simulink model "inverter_switching_StudentVersion"  (R2025a)
settings: Solver=VariableStepAuto  StartTime=0.0  StopTime=0.2  MaxStep=1e-6  RelTol=1e-3
values from neighbouring files (symbols this model uses):
  C_Filter = 300e-6    (= 0.0003)    [parameters_StudentVersion.m]
  Fref = 50    [parameters_StudentVersion.m]
  kFilterIdq = wnFiltreIdq/WnIdq    (= 1)    [parameters_StudentVersion.m]
  kFilterVdq = wnFiltreVdq/WnVdq    (= 1)    [parameters_StudentVersion.m]
  L_Filter = 1e-3    (= 0.001)    [parameters_StudentVersion.m]
  rL_filter = 0.1    [parameters_StudentVersion.m]
  T32 = sqrt(2/3)*[1 0; -1/2 sqrt(3)/2; -1/2 -sqrt(3)/2]    [parameters_StudentVersion.m]
  Ts = 1/Fs    (= 5e-05)    [parameters_StudentVersion.m]
  Vdc = 800    [parameters_StudentVersion.m]
  VrmsRef = 40    [parameters_StudentVersion.m]
  WnIdq = 12000    [parameters_StudentVersion.m]
  WnVdq = 1200    [parameters_StudentVersion.m]
  zeta = 1/sqrt(2)    [parameters_StudentVersion.m]
undefined symbols (not defined in the file or in its folder): DiscIntNeverNeededParam
libraries: nesl_utility x18, ee_lib x15, fl_lib x12, simulink x5
(part 2 of 2)

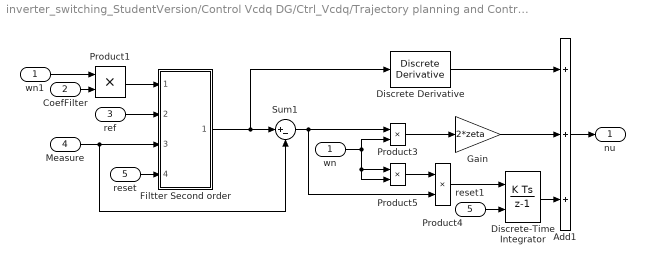
== system inverter_switching_StudentVersion/Control Vcdq DG/Ctrl_Vcdq/Trajectory planning and Control 1 ==
  wn : Inport
  CoefFilter : Inport  Port=2
  ref : Inport  Port=3
  Measure : Inport  Port=4
  reset : Inport  Port=5
  Add1 : Sum  Inputs=+++
  Discrete Derivative : simulink/Discrete/Discrete Derivative  gainval=1.0  ICPrevScaledInput=0.0  OutMin=[]  OutMax=[]  OutDataType=fixdt(1, 16)  OutScaling=2^-10  DoSatur=off
  Discrete-Time Integrator : DiscreteIntegrator  ExternalReset=level  SampleTime=-1  ICPrevOutput=DiscIntNeverNeededParam  ICPrevScaledInput=DiscIntNeverNeededParam
  Filtter Second order : Subsystem
  Gain : Gain  Gain=2*zeta
  Product{1,3..5} (4 alike) : Product
  Sum1 : Sum  Inputs=|+-
  reset1 : InportShadow  Port=5
  wn1 : InportShadow
  nu : Outport
  wires:
  Add1/1 -> nu/1
  CoefFilter/1 -> Product1/2
  Measure/1 -> Filtter Second order/3(init1), Sum1/2
  ref/1 -> Filtter Second order/2(yref1)
  wn1/1 -> Product1/1
  Product1/1 -> Filtter Second order/1(wfilter1)
  Filtter Second order/1(yref_filtre 1) -> Discrete Derivative/1, Sum1/1
  Gain/1 -> Add1/2
  Discrete-Time Integrator/1 -> Add1/3
  Product3/1 -> Gain/1
  wn/1 -> Product3/2, Product5/1, Product5/2
  Product5/1 -> Product4/1
  Product4/1 -> Discrete-Time Integrator/1
  Sum1/1 -> Product3/1, Product4/2
  reset/1 -> Filtter Second order/4(reset)
  reset1/1 -> Discrete-Time Integrator/2
  Discrete Derivative/1 -> Add1/1

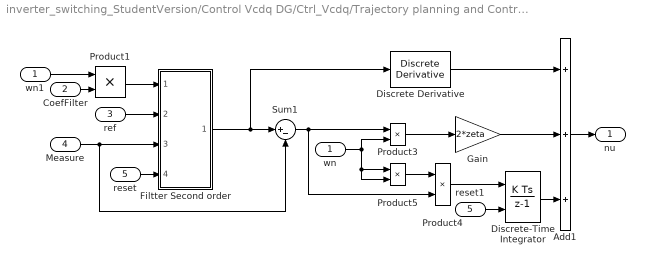
== system inverter_switching_StudentVersion/Control Vcdq DG/Ctrl_Vcdq/Trajectory planning and Control 2 ==
  wn : Inport
  CoefFilter : Inport  Port=2
  ref : Inport  Port=3
  Measure : Inport  Port=4
  reset : Inport  Port=5
  Add1 : Sum  Inputs=+++
  Discrete Derivative : simulink/Discrete/Discrete Derivative  gainval=1.0  ICPrevScaledInput=0.0  OutMin=[]  OutMax=[]  OutDataType=fixdt(1, 16)  OutScaling=2^-10  DoSatur=off
  Discrete-Time Integrator : DiscreteIntegrator  ExternalReset=level  SampleTime=-1  ICPrevOutput=DiscIntNeverNeededParam  ICPrevScaledInput=DiscIntNeverNeededParam
  Filtter Second order : Subsystem
  Gain : Gain  Gain=2*zeta
  Product{1,3..5} (4 alike) : Product
  Sum1 : Sum  Inputs=|+-
  reset1 : InportShadow  Port=5
  wn1 : InportShadow
  nu : Outport
  wires:
  reset1/1 -> Discrete-Time Integrator/2
  reset/1 -> Filtter Second order/4(reset)
  Sum1/1 -> Product4/2, Product3/1
  Product4/1 -> Discrete-Time Integrator/1
  Product5/1 -> Product4/1
  wn/1 -> Product5/2, Product5/1, Product3/2
  Product3/1 -> Gain/1
  Discrete-Time Integrator/1 -> Add1/3
  Gain/1 -> Add1/2
  Filtter Second order/1(yref_filtre 1) -> Discrete Derivative/1, Sum1/1
  Product1/1 -> Filtter Second order/1(wfilter1)
  wn1/1 -> Product1/1
  ref/1 -> Filtter Second order/2(yref1)
  Measure/1 -> Sum1/2, Filtter Second order/3(init1)
  CoefFilter/1 -> Product1/2
  Add1/1 -> nu/1
  Discrete Derivative/1 -> Add1/1

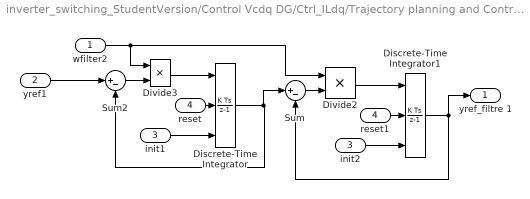
== system inverter_switching_StudentVersion/Control Vcdq DG/Ctrl_ILdq/Trajectory planning and Control 1/Filtter Second order ==
  wfilter2 : Inport
  yref1 : Inport  Port=2
  init1 : Inport  Port=3
  reset : Inport  Port=4
  Discrete-Time Integrator : DiscreteIntegrator  ExternalReset=level  InitialConditionSource=external  SampleTime=-1  ICPrevOutput=DiscIntNeverNeededParam  ICPrevScaledInput=DiscIntNeverNeededParam
  Discrete-Time Integrator1 : DiscreteIntegrator  ExternalReset=level  InitialConditionSource=external  SampleTime=-1  ICPrevOutput=DiscIntNeverNeededParam  ICPrevScaledInput=DiscIntNeverNeededParam
  Divide2 : Product  Inputs=**
  Divide3 : Product  Inputs=**
  Sum : Sum  Inputs=|+-
  Sum2 : Sum  Inputs=|+-
  init2 : InportShadow  Port=3
  reset1 : InportShadow  Port=4
  yref_filtre 1 : Outport
  wires:
  reset1/1 -> Discrete-Time Integrator1/2
  reset/1 -> Discrete-Time Integrator/2
  init2/1 -> Discrete-Time Integrator1/3
  Sum2/1 -> Divide3/2
  Discrete-Time Integrator1/1 -> yref_filtre 1/1, Sum/2
  yref1/1 -> Sum2/1
  Sum/1 -> Divide2/2
  Divide3/1 -> Discrete-Time Integrator/1
  Discrete-Time Integrator/1 -> Sum/1, Sum2/2
  init1/1 -> Discrete-Time Integrator/3
  wfilter2/1 -> Divide3/1, Divide2/1
  Divide2/1 -> Discrete-Time Integrator1/1

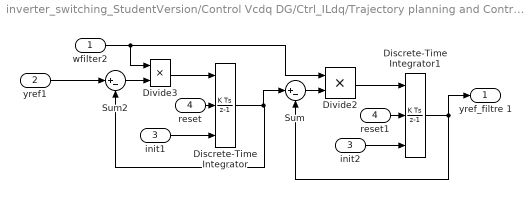
== system inverter_switching_StudentVersion/Control Vcdq DG/Ctrl_ILdq/Trajectory planning and Control 2/Filtter Second order ==
  wfilter2 : Inport
  yref1 : Inport  Port=2
  init1 : Inport  Port=3
  reset : Inport  Port=4
  Discrete-Time Integrator : DiscreteIntegrator  ExternalReset=level  InitialConditionSource=external  SampleTime=-1  ICPrevOutput=DiscIntNeverNeededParam  ICPrevScaledInput=DiscIntNeverNeededParam
  Discrete-Time Integrator1 : DiscreteIntegrator  ExternalReset=level  InitialConditionSource=external  SampleTime=-1  ICPrevOutput=DiscIntNeverNeededParam  ICPrevScaledInput=DiscIntNeverNeededParam
  Divide2 : Product  Inputs=**
  Divide3 : Product  Inputs=**
  Sum : Sum  Inputs=|+-
  Sum2 : Sum  Inputs=|+-
  init2 : InportShadow  Port=3
  reset1 : InportShadow  Port=4
  yref_filtre 1 : Outport
  wires:
  Divide2/1 -> Discrete-Time Integrator1/1
  wfilter2/1 -> Divide2/1, Divide3/1
  init1/1 -> Discrete-Time Integrator/3
  Discrete-Time Integrator/1 -> Sum2/2, Sum/1
  Divide3/1 -> Discrete-Time Integrator/1
  Sum/1 -> Divide2/2
  yref1/1 -> Sum2/1
  Discrete-Time Integrator1/1 -> Sum/2, yref_filtre 1/1
  Sum2/1 -> Divide3/2
  init2/1 -> Discrete-Time Integrator1/3
  reset/1 -> Discrete-Time Integrator/2
  reset1/1 -> Discrete-Time Integrator1/2

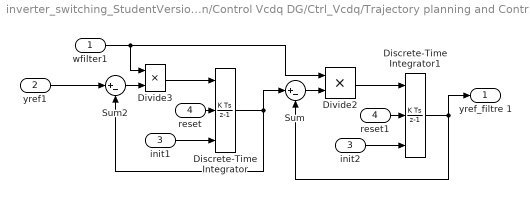
== system inverter_switching_StudentVersion/Control Vcdq DG/Ctrl_Vcdq/Trajectory planning and Control 1/Filtter Second order ==
  wfilter1 : Inport
  yref1 : Inport  Port=2
  init1 : Inport  Port=3
  reset : Inport  Port=4
  Discrete-Time Integrator : DiscreteIntegrator  ExternalReset=level  InitialConditionSource=external  SampleTime=-1  ICPrevOutput=DiscIntNeverNeededParam  ICPrevScaledInput=DiscIntNeverNeededParam
  Discrete-Time Integrator1 : DiscreteIntegrator  ExternalReset=level  InitialConditionSource=external  SampleTime=-1  ICPrevOutput=DiscIntNeverNeededParam  ICPrevScaledInput=DiscIntNeverNeededParam
  Divide2 : Product  Inputs=**
  Divide3 : Product  Inputs=**
  Sum : Sum  Inputs=|+-
  Sum2 : Sum  Inputs=|+-
  init2 : InportShadow  Port=3
  reset1 : InportShadow  Port=4
  yref_filtre 1 : Outport
  wires:
  Divide2/1 -> Discrete-Time Integrator1/1
  wfilter1/1 -> Divide2/1, Divide3/1
  init1/1 -> Discrete-Time Integrator/3
  Discrete-Time Integrator/1 -> Sum/1, Sum2/2
  Divide3/1 -> Discrete-Time Integrator/1
  Sum/1 -> Divide2/2
  yref1/1 -> Sum2/1
  Discrete-Time Integrator1/1 -> Sum/2, yref_filtre 1/1
  Sum2/1 -> Divide3/2
  init2/1 -> Discrete-Time Integrator1/3
  reset/1 -> Discrete-Time Integrator/2
  reset1/1 -> Discrete-Time Integrator1/2

== system inverter_switching_StudentVersion/Control Vcdq DG/Ctrl_Vcdq/Trajectory planning and Control 2/Filtter Second order ==
  wfilter1 : Inport
  yref1 : Inport  Port=2
  init1 : Inport  Port=3
  reset : Inport  Port=4
  Discrete-Time Integrator : DiscreteIntegrator  ExternalReset=level  InitialConditionSource=external  SampleTime=-1  ICPrevOutput=DiscIntNeverNeededParam  ICPrevScaledInput=DiscIntNeverNeededParam
  Discrete-Time Integrator1 : DiscreteIntegrator  ExternalReset=level  InitialConditionSource=external  SampleTime=-1  ICPrevOutput=DiscIntNeverNeededParam  ICPrevScaledInput=DiscIntNeverNeededParam
  Divide2 : Product  Inputs=**
  Divide3 : Product  Inputs=**
  Sum : Sum  Inputs=|+-
  Sum2 : Sum  Inputs=|+-
  init2 : InportShadow  Port=3
  reset1 : InportShadow  Port=4
  yref_filtre 1 : Outport
  wires:
  reset1/1 -> Discrete-Time Integrator1/2
  reset/1 -> Discrete-Time Integrator/2
  init2/1 -> Discrete-Time Integrator1/3
  Sum2/1 -> Divide3/2
  Discrete-Time Integrator1/1 -> yref_filtre 1/1, Sum/2
  yref1/1 -> Sum2/1
  Sum/1 -> Divide2/2
  Divide3/1 -> Discrete-Time Integrator/1
  Discrete-Time Integrator/1 -> Sum/1, Sum2/2
  init1/1 -> Discrete-Time Integrator/3
  wfilter1/1 -> Divide3/1, Divide2/1
  Divide2/1 -> Discrete-Time Integrator1/1

== matlab function inverter_switching_StudentVersion/Control Vcdq DG/Ctrl_ILdq/MATLAB Function ==
  data: nuId input; VdRef output; nuIq input; Omega input; ILd input; ILq input; Vcd input; Vcq input; VqRef output; L_DG parameter; rL_DG parameter
function [VdRef,VqRef] = fcn(nuId,nuIq,Omega,ILd,ILq,Vcd,Vcq,L_DG, rL_DG)

    VdRef= L_DG*nuId+rL_DG*ILd+Vcd-L_DG*Omega*ILq;
    VqRef= L_DG*nuIq+rL_DG*ILq+Vcq+L_DG*Omega*ILd;
end

== matlab function inverter_switching_StudentVersion/Control Vcdq DG/Ctrl_Vcdq/MATLAB Function ==
  data: nuVd input; IdRef output; nuVq input; Omega input; ILined input; ILineq input; Vcd input; Vcq input; IqRef output; C_DG parameter
function [IdRef,IqRef] = fcn(nuVd,nuVq,Omega,ILined,ILineq,Vcd,Vcq,C_DG)

IdRef = C_DG*nuVd+ILined-C_DG*Omega*Vcq;
IqRef = C_DG*nuVq+ILineq+C_DG*Omega*Vcd;
end
